simulink model "Count_with_While_Loop"  (R2016b)
settings: Solver=VariableStepAuto  StartTime=0.0  StopTime=10.0  RelTol=1e-3
settings Model: Creator=Saher Ghanem  LastModifiedBy=Saher Ghanem

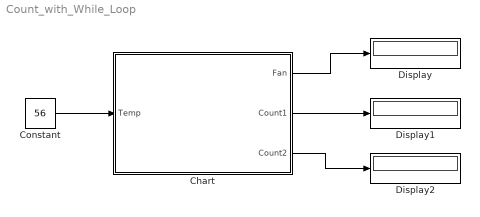
== system Count_with_While_Loop ==
  Chart : Stateflow chart  TreatAsAtomicUnit=on
  Constant : Constant  Value=56
  Display : Display
  Display1 : Display
  Display2 : Display
  wires:
  Constant/1 -> Chart/1(Temp)
  Chart/1(Fan) -> Display/1
  Chart/2(Count1) -> Display1/1
  Chart/3(Count2) -> Display2/1

== stateflow chart Count_with_While_Loop/Chart ==
  (default) -> (junction 28) : /* While */
  (junction 28) -> (junction 30)
  (junction 30) -> (junction 29) [order 1] : [Count1<5]
  (junction 29) -> (junction 31) : {Count1=Count1+1;}
  (junction 31) -> (junction 30)
  (junction 30) -> (junction 32) [order 2]
  data: Temp input double; Fan output double; Count1 output double; Count2 output double
